simulink model "pruebasAPF"  (R2023b)
settings: Solver=VariableStepAuto  StartTime=0.0  StopTime=inf  RelTol=1e-3
values from neighbouring files (symbols this model uses):
  resultante = cat(3, px,py)    [graficar_nube.m]
undefined symbols (not defined in the file or in its folder): Standard_Devices, UDP_Protocol
libraries: sldrtlib x4
settings Model: Creator=eduar  LastModifiedBy=eduar

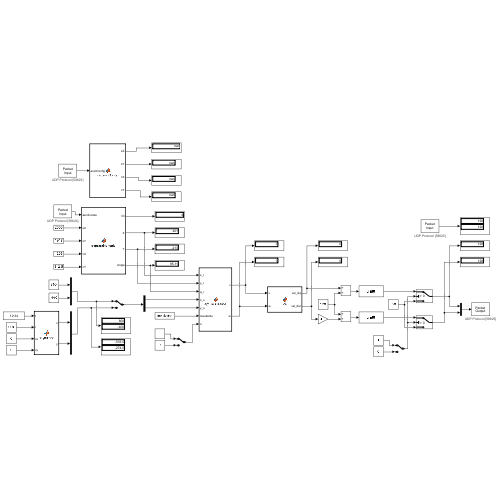
[thumbnail: Simulink's stored preview of the top-level diagram]
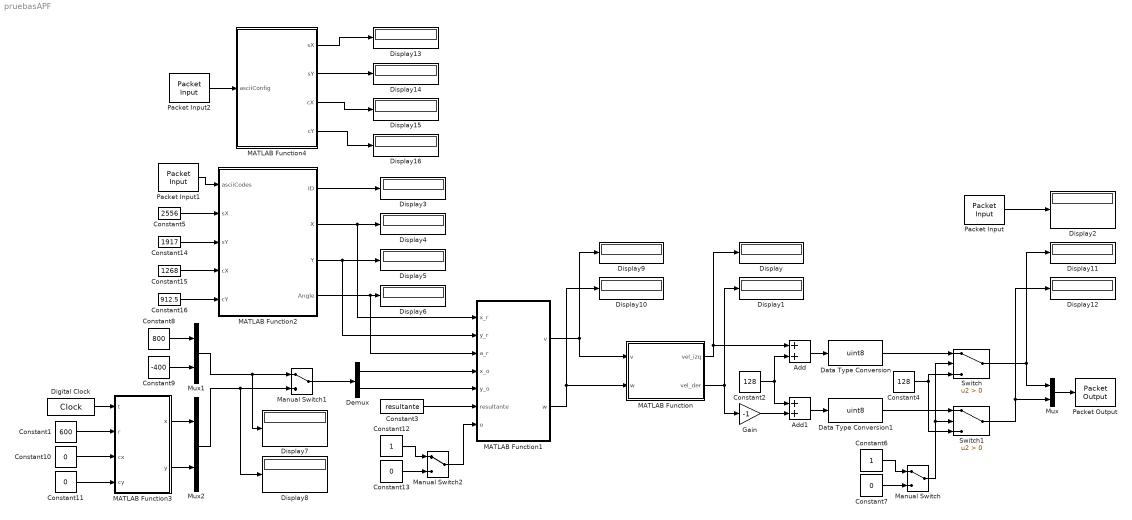
== system pruebasAPF ==
  Add : Sum
  Add1 : Sum
  Constant1 : Constant  Value=600
  Constant{7,10..11,13} (4 alike) : Constant  Value=0
  Constant12 : Constant
  Constant14 : Constant  Value=1917
  Constant15 : Constant  Value=1268
  Constant16 : Constant  Value=912.5
  Constant2 : Constant  Value=128
  Constant3 : Constant  Value=resultante
  Constant4 : Constant  Value=128
  Constant5 : Constant  Value=2556
  Constant6 : Constant
  Constant8 : Constant  Value=800
  Constant9 : Constant  Value=-400
  Data Type Conversion : DataTypeConversion  OutDataTypeStr=uint8  SaturateOnIntegerOverflow=off  RndMeth=Floor
  Data Type Conversion1 : DataTypeConversion  OutDataTypeStr=uint8  SaturateOnIntegerOverflow=off  RndMeth=Floor
  Demux : Demux  Outputs=2
  Digital Clock : DigitalClock
  Display{,1..16} (17 alike) : Display
      Display10 settings: Decimation=2
      Display13 settings: Decimation=2
      Display14 settings: Decimation=2
      Display15 settings: Decimation=2
      Display16 settings: Decimation=2
      Display3 settings: Decimation=2
      Display4 settings: Decimation=2
      Display5 settings: Decimation=2
      Display6 settings: Decimation=2
      Display7 settings: Decimation=2
      Display8 settings: Decimation=2
      Display9 settings: Decimation=2
  Gain : Gain  Gain=-1
  MATLAB Function : MATLAB Function  TreatAsAtomicUnit=on
  MATLAB Function1 : MATLAB Function  TreatAsAtomicUnit=on
  MATLAB Function2 : MATLAB Function  TreatAsAtomicUnit=on
  MATLAB Function3 : MATLAB Function  TreatAsAtomicUnit=on
  MATLAB Function4 : MATLAB Function  TreatAsAtomicUnit=on
  Manual Switch : ManualSwitch
  Manual Switch1 : ManualSwitch
  Manual Switch2 : ManualSwitch
  Mux : Mux  Inputs=2
  Mux1 : Mux  Inputs=2
  Mux2 : Mux  Inputs=2
  Packet Input : sldrtlib/Packet Input  SampleTime=1  MaxMissedTicks=inf  ShowMissedTicks=off  YieldWhenWaiting=off  DrvName=Standard_Devices/UDP_Protocol  DrvAddress=58625  DrvOptions=[0 58625 49 57 50 46 49 54 56 46 49 51 55 46 49 56 55 0 0 0 0 0 0 0 0 0 0 0 0 0 0 0 0 0 0 0 0 0 0 0 0 0 0 0 0 0 0 0 0 0 0 0 0 0 0 0 0 0 0 0 0 0 0 0 0 0 0 0 0 0 0 0 0 0 0 0 0 0 0 0 0 0 0 0 0 0 0 0 0 0 0 0 0 0 0 0 0 0 0 0 0 0 0 0 0 0 0 0 0 0 0 0 0 0 0 0 0 0 0 0 0 0 0 0 0 0 0 0 0 0 0 0 0 0 0 0 0 0 0 0 0 0 0 0 0 0 0 0 0 0 0 0 0 0 0 0 0 0 0 0 0 0 0 0 0 0 0 0 0 0 0 0 0 0 0 0 0 0 0 0 0 0 0 0 0 0 0 0 0 0 0 0 0 0 0 0 0 0 0 0 0 0 0 0 0 0 0 0 0 0 0 0 0 0 0 0 0 0 0 0 0 0 0 0 0 0 0 0 0 0 0 0 0 0 0 0 0 0 0 0 0 0 0 0 0 0 0 0 0 0 0 0 0 0 0 0]  PacketSize=2  DataTypes='2*uint8'  ShowReady=off  ShowError=off  PacketID=1  ByteOrder=1  ShowTimestamp=off
      settings: AttributesFormatString=UDP Protocol [58625]
  Packet Input1 : sldrtlib/Packet Input  SampleTime=0.01  MaxMissedTicks=inf  ShowMissedTicks=off  YieldWhenWaiting=off  DrvName=Standard_Devices/UDP_Protocol  DrvAddress=58624  DrvOptions=[0 58624 49 50 55 46 48 46 48 46 49 0 0 0 0 0 0 0 0 0 0 0 0 0 0 0 0 0 0 0 0 0 0 0 0 0 0 0 0 0 0 0 0 0 0 0 0 0 0 0 0 0 0 0 0 0 0 0 0 0 0 0 0 0 0 0 0 0 0 0 0 0 0 0 0 0 0 0 0 0 0 0 0 0 0 0 0 0 0 0 0 0 0 0 0 0 0 0 0 0 0 0 0 0 0 0 0 0 0 0 0 0 0 0 0 0 0 0 0 0 0 0 0 0 0 0 0 0 0 0 0 0 0 0 0 0 0 0 0 0 0 0 0 0 0 0 0 0 0 0 0 0 0 0 0 0 0 0 0 0 0 0 0 0 0 0 0 0 0 0 0 0 0 0 0 0 0 0 0 0 0 0 0 0 0 0 0 0 0 0 0 0 0 0 0 0 0 0 0 0 0 0 0 0 0 0 0 0 0 0 0 0 0 0 0 0 0 0 0 0 0 0 0 0 0 0 0 0 0 0 0 0 0 0 0 0 0 0 0 0 0 0 0 0 0 0 0 0 0 0 0 0 0 0 0 0]  PacketSize=24  DataTypes='24*int8'  ShowReady=off  ShowError=off  PacketID=1  ByteOrder=1  ShowTimestamp=off
      settings: AttributesFormatString=UDP Protocol [58624]
  Packet Input2 : sldrtlib/Packet Input  SampleTime=0.01  MaxMissedTicks=inf  ShowMissedTicks=off  YieldWhenWaiting=off  DrvName=Standard_Devices/UDP_Protocol  DrvAddress=58623  DrvOptions=[0 58623 49 50 55 46 48 46 48 46 50 0 0 0 0 0 0 0 0 0 0 0 0 0 0 0 0 0 0 0 0 0 0 0 0 0 0 0 0 0 0 0 0 0 0 0 0 0 0 0 0 0 0 0 0 0 0 0 0 0 0 0 0 0 0 0 0 0 0 0 0 0 0 0 0 0 0 0 0 0 0 0 0 0 0 0 0 0 0 0 0 0 0 0 0 0 0 0 0 0 0 0 0 0 0 0 0 0 0 0 0 0 0 0 0 0 0 0 0 0 0 0 0 0 0 0 0 0 0 0 0 0 0 0 0 0 0 0 0 0 0 0 0 0 0 0 0 0 0 0 0 0 0 0 0 0 0 0 0 0 0 0 0 0 0 0 0 0 0 0 0 0 0 0 0 0 0 0 0 0 0 0 0 0 0 0 0 0 0 0 0 0 0 0 0 0 0 0 0 0 0 0 0 0 0 0 0 0 0 0 0 0 0 0 0 0 0 0 0 0 0 0 0 0 0 0 0 0 0 0 0 0 0 0 0 0 0 0 0 0 0 0 0 0 0 0 0 0 0 0 0 0 0 0 0 0]  PacketSize=24  DataTypes='24*int8'  ShowReady=off  ShowError=off  PacketID=1  ByteOrder=1  ShowTimestamp=off
      settings: AttributesFormatString=UDP Protocol [58623]
  Packet Output : sldrtlib/Packet Output  SampleTime=1  MaxMissedTicks=inf  ShowMissedTicks=off  YieldWhenWaiting=off  DrvName=Standard_Devices/UDP_Protocol  DrvAddress=58625  DrvOptions=[0 58625 49 57 50 46 49 54 56 46 49 51 55 46 49 56 55 0 0 0 0 0 0 0 0 0 0 0 0 0 0 0 0 0 0 0 0 0 0 0 0 0 0 0 0 0 0 0 0 0 0 0 0 0 0 0 0 0 0 0 0 0 0 0 0 0 0 0 0 0 0 0 0 0 0 0 0 0 0 0 0 0 0 0 0 0 0 0 0 0 0 0 0 0 0 0 0 0 0 0 0 0 0 0 0 0 0 0 0 0 0 0 0 0 0 0 0 0 0 0 0 0 0 0 0 0 0 0 0 0 0 0 0 0 0 0 0 0 0 0 0 0 0 0 0 0 0 0 0 0 0 0 0 0 0 0 0 0 0 0 0 0 0 0 0 0 0 0 0 0 0 0 0 0 0 0 0 0 0 0 0 0 0 0 0 0 0 0 0 0 0 0 0 0 0 0 0 0 0 0 0 0 0 0 0 0 0 0 0 0 0 0 0 0 0 0 0 0 0 0 0 0 0 0 0 0 0 0 0 0 0 0 0 0 0 0 0 0 0 0 0 0 0 0 0 0 0 0 0 0 0 0 0 0 0 0]  PacketSize=2  DataTypes='2*uint8'  ShowReady=off  ShowError=off  PacketID=1  ByteOrder=1  InitialValue=[]  FinalValue=[]
      settings: AttributesFormatString=UDP Protocol [58625]
  Switch : Switch  Criteria=u2 > Threshold  SaturateOnIntegerOverflow=off  InputSameDT=off
  Switch1 : Switch  Criteria=u2 > Threshold  SaturateOnIntegerOverflow=off  InputSameDT=off
  wires:
  MATLAB Function/2(vel_der) -> Display1/1, Gain/1
  MATLAB Function/1(vel_izq) -> Display/1, Add/1
  Mux/1 -> Packet Output/1
  Add/1 -> Data Type Conversion/1
  Add1/1 -> Data Type Conversion1/1
  Constant4/1 -> Switch/3, Switch1/3
  Manual Switch/1 -> Switch/2, Switch1/2
  Data Type Conversion1/1 -> Switch1/1
  Data Type Conversion/1 -> Switch/1
  Constant6/1 -> Manual Switch/1
  Constant7/1 -> Manual Switch/2
  Switch1/1 -> Display12/1, Mux/2
  Switch/1 -> Mux/1, Display11/1
  Packet Input/1 -> Display2/1
  MATLAB Function2/1(ID) -> Display3/1
  Packet Input1/1 -> MATLAB Function2/1(asciiCodes)
  Digital Clock/1 -> MATLAB Function3/1(t)
  Constant1/1 -> MATLAB Function3/2(r)
  Constant10/1 -> MATLAB Function3/3(cx)
  Constant11/1 -> MATLAB Function3/4(cy)
  MATLAB Function3/1(x) -> Mux2/1
  MATLAB Function3/2(y) -> Mux2/2
  Manual Switch1/1 -> Demux/1
  Mux1/1 -> Display7/1, Manual Switch1/1
  Mux2/1 -> Display8/1, Manual Switch1/2
  Gain/1 -> Add1/2
  Constant2/1 -> Add/2, Add1/1
  MATLAB Function2/4(Angle) -> MATLAB Function1/3(a_r), Display6/1
  MATLAB Function2/3(Y) -> Display5/1, MATLAB Function1/2(y_r)
  MATLAB Function2/2(X) -> Display4/1, MATLAB Function1/1(x_r)
  Constant8/1 -> Mux1/1
  Constant9/1 -> Mux1/2
  Demux/1 -> MATLAB Function1/4(x_o)
  Demux/2 -> MATLAB Function1/5(y_o)
  MATLAB Function4/2(sY) -> Display14/1
  MATLAB Function4/1(sX) -> Display13/1
  MATLAB Function1/1(v) -> MATLAB Function/1(v), Display9/1
  MATLAB Function1/2(w) -> MATLAB Function/2(w), Display10/1
  Constant12/1 -> Manual Switch2/1
  Constant13/1 -> Manual Switch2/2
  Manual Switch2/1 -> MATLAB Function1/7(o)
  Packet Input2/1 -> MATLAB Function4/1(asciiConfig)
  MATLAB Function4/3(cX) -> Display15/1
  MATLAB Function4/4(cY) -> Display16/1
  Constant3/1 -> MATLAB Function1/6(resultante)
  Constant5/1 -> MATLAB Function2/2(sX)
  Constant16/1 -> MATLAB Function2/5(cY)
  Constant15/1 -> MATLAB Function2/4(cX)
  Constant14/1 -> MATLAB Function2/3(sY)

== matlab function pruebasAPF/MATLAB Function1 ==
  data: x_r input; v output; y_r input; a_r input; x_o input; y_o input; resultante input; o input; w output
function [v, w] = apf_resultante(x_r, y_r, a_r, x_o, y_o, resultante, o)
    rp = 30; % Radio de protección [mm]
    ap = 5; % Ángulo de protección [°]
    
    if o == 1 %% En caso de que se desee seguir el comportamiento 
        kv = 220; % Constante velocidad lineal
        kw = 0.05; % Constante velocidad angular

        kapf = 8; % Constante de la escala del APF
        dapf = sqrt((y_o-y_r)^2 + (x_o-x_r)^2);
        ra = 400; % Radio de acción del campo 
        
        if dapf <= ra
            % Obtener las coordenadas en la matriz resultante
            x_idx = round(50+(x_r - x_o)/kapf); % Índice x en la matriz
            y_idx = round(50+(y_r - y_o)/kapf); % Índice y en la matriz

            if x_idx>0 && x_idx<101 && y_idx>0 && y_idx<101
                % Obtener las magnitudes de los vectores en las direcciones x e y
                mag_x = resultante(x_idx, y_idx, 1);
                mag_y = resultante(x_idx, y_idx, 2);
            else
                mag_x = 0;
                mag_y = 0;
            end
            
            % Calcular la velocidad lineal
            v = kv * sqrt(mag_x^2 + mag_y^2);
    
            % Calcular el ángulo del vector en la matriz resultante
            a_o = 90 + atan2d(mag_y, mag_x); % Utilizar atan2d para obtener el ángulo en grados
            
            % Diferencia entre la orientación del robot y la deseada
            da_obj = a_o - a_r;
            
            % Ajuste de ángulo entre -180 y 180
            if da_obj > 180
                da_obj = da_obj - 360;
            elseif da_obj < -180
                da_obj = da_obj + 360;
            end
            
            % Calcular la velocidad angular
            w = kw * da_obj;
            
            % Aplicar condiciones de protección
            if sqrt(x_r^2 + y_r^2) < rp
                v = 0;
            end
            if abs(da_obj) < ap
                w = 0;
            end
    
        else
            v = 0;
            w = 0;
        end
    elseif o == 0 %% Para llevar al robot a unas coordenadas objetivo
        kv = 0.8; % Constante velocidad lineal
        kw = 0.05; % Constante velocidad angular

        % Distancia del robot al objetivo
        d_obj = sqrt((x_o-x_r)^2 + (y_o-y_r)^2);
    
        % Cálculo de velocidad lineal
        v = kv * d_obj;
        
        % Ángulo con respecto al eje x del robot al objetivo
        a_o = atan2d(y_o-y_r, x_o-x_r) - 90; % Utilizar atan2d para obtener el ángulo en grados
        if a_o < 0
            a_o = a_o + 360;
        end
    
        % Diferencia entre orientación del robot y deseada
        da_obj = a_o - a_r;
    
        % Ajuste de ángulo entre -180 y 180
        if da_obj > 180
            da_obj = da_obj - 360;
        elseif da_obj < -180
            da_obj = da_obj + 360;
        end
    
        % Cálculo de velocidad angular
        w = kw * da_obj;
    
        if (d_obj < rp)
            v = 0;
        end
        if (abs(da_obj) < ap)
            w = 0;
        end
    else
        v = 0;
        w = 0;
    end 
end

== matlab function pruebasAPF/MATLAB Function ==
  data: vel_izq output; v input; vel_der output; w input
function [vel_izq, vel_der] = fcn(v, w)
    % Parametros Robot
    r = 30; % Radio de las llantas [mm]
    b = 85; % Distancia de P a las llantas en y1 [mm]
    d = 60; % Distancia de P a las llantas en x1 [mm]

    % Verificar si v o w son "nan"
    if isnan(v) || isnan(w)
        % Si v o w son "nan", asignar 0 a ambas velocidades
        vel_der = 0;
        vel_izq = 0;
    else
        % Cálculo de las velocidades de giro de las llantas
        vLlantaDer = (v + b*w)/r; % Vel de llanta derecha
        vLlantaIzq = (v - b*w)/r; % Vel de llanta izquierda

        velMax = 100; % Velocidad máxima
        % Límite de la velocidad máxima
        if (vLlantaDer > velMax)
            vLlantaDer = velMax;
        elseif (vLlantaDer < -velMax)
            vLlantaDer = -velMax;
        end

        if (vLlantaIzq > velMax)
            vLlantaIzq = velMax;
        elseif (vLlantaIzq < -velMax)
            vLlantaIzq = -velMax;
        end

        vel_der = vLlantaDer;
        vel_izq = vLlantaIzq;
    end
end

== matlab function pruebasAPF/MATLAB Function2 ==
  data: ID output; asciiCodes input; X output; Y output; Angle output; sX input; sY input; cX input; cY input
function [ID, X, Y, Angle] = separarMensaje(asciiCodes, sX, sY, cX, cY)
    % Convertir los códigos ASCII a caracteres
    asciiChars = char(asciiCodes);

    % Definir índices fijos para separar la cadena
    commaIndices = [7, 13, 19];

    % Extraer las partes de la cadena basadas en índices fijos
    ID = str2double(asciiChars(2:commaIndices(1)));
    X = real(str2double(asciiChars(commaIndices(1)+1:commaIndices(2))));
    Y = real(str2double(asciiChars(commaIndices(2)+1:commaIndices(3))));
    Angle = real(str2double(asciiChars(commaIndices(3)+1:end)));

    X = round(real(X*(sX/1000) - cX));
    Y = round(real(Y*(sY/1000) - cY));
    Angle = real(Angle*(360/(2*pi))*(1/1000));
end

== matlab function pruebasAPF/MATLAB Function3 ==
  data: x output; t input; y output; r input; cx input; cy input
function [x,y] = trayectoria(t, r, cx, cy)
    x = r*cos(t/10)+cx;
    y = r*sin(t/10)+cy;
end

== matlab function pruebasAPF/MATLAB Function4 ==
  data: sX output; asciiConfig input; sY output; cX output; cY output
function [sX, sY, cX, cY] = separarConfig(asciiConfig)
    % Convertir los códigos ASCII a caracteres
    asciiC = char(asciiConfig);

    % Definir índices fijos para separar la cadena
    commaIndices = [7, 13, 19];

    % Extraer las partes de la cadena basadas en índices fijos
    sX = str2double(asciiC(2:commaIndices(1)-1));
    sY = real(str2double(asciiC(commaIndices(1)+1:commaIndices(2)-1)));
    cX = real(str2double(asciiC(commaIndices(2)+1:commaIndices(3)-1)));
    cY = real(str2double(asciiC(commaIndices(3)+1:end)));

    cX = real(cX *(sX/1000));
    cY = real(cY *(sY/1000));
end
